simulink model "data_acq_passiveV2"  (R2016b)
settings: Solver=FixedStepDiscrete  StartTime=0.0  StopTime=300  FixedStep=.001  RelTol=1e-3  EnableMultiTasking=on
values from neighbouring files (symbols this model uses):
  offset = [0 0]    [Calibration_Run_Script.m]    (also in DAQ_Run_Script.m; bias.m = signal)
undefined symbols (not defined in the file or in its folder): bit, fdesignblkfcn, gcbh, Standard
libraries: slrtlib x11, xpclib x6, canmsglib x5, simulink x5, xpcnilib x3
(part 2 of 2)

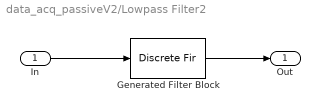
== system data_acq_passiveV2/Lowpass Filter2 ==
  In : Inport
  Generated Filter Block : DiscreteFir  Tag=BlockMethodSubSystem  Coefficients=[0.0035257793515495774 0.0038119531647798038 0.0041036148788394806 0.0044003780267683791 0.0047018389448218933 0.0050075775498282637 0.0053171581667394901 0.0056301304044040169 0.0059460300774376931 0.0062643801719234971 0.0065846918525311708 0.0069064655085147161 0.0072291918359202803 0.0075523529532183957 0.0078754235474644951 0.0081978720479896055 0.008519161824529782 0.008838752406618456 0.0091561007209909322 0.0094706623436844779 0.0097818927634617959 0.010089248653139572 0.010392189145368247 0.010690177109383412 0.010982680425234054 0.011269173251988259 0.011549137286422439 0.011822063008716528 0.012087450911703952 0.012344812710262444 0.01259367252747858 0.012833568054276996 0.013064051679271809 0.013284691585675896 0.013495072812189788 0.013694798274888394 0.013883489747229208 0.014060788795419015 0.014226357666499202 0.014379880126639598 0.014521062247269227 0.014649633136817507 0.014765345615991476 0.014867976834673335 0.014957328828686459 0.015033229014848307 0.015095530622902396 0.015144113063101152 0.015178882228393269 0.015199770730355538 0.015206738068197194 0.015199770730355538 0.015178882228393269 0.015144113063101152 0.015095530622902396 0.015033229014848307 0.014957328828686459 0.014867976834673335 0.014765345615991476 0.014649633136817507 0.014521062247269227 0.014379880126639598 0.014226357666499202 0.014060788795419015 0.013883489747229208 0.013694798274888394 0.013495072812189788 0.013284691585675896 0.013064051679271809 0.012833568054276996 0.01259367252747858 0.012344812710262444 0.012087450911703952 0.011822063008716528 0.011549137286422439 0.011269173251988259 0.010982680425234054 0.010690177109383412 0.010392189145368247 0.010089248653139572 0.0097818927634617959 0.0094706623436844779 0.0091561007209909322 0.008838752406618456 0.008519161824529782 0.0081978720479896055 0.0078754235474644951 0.0075523529532183957 0.0072291918359202803 0.0069064655085147161 0.0065846918525311708 0.0062643801719234971 0.0059460300774376931 0.0056301304044040169 0.0053171581667394901 0.0050075775498282637 0.0047018389448218933 0.0044003780267683791 0.0041036148788394806 0.0038119531647798038 0.0035257793515495774]  InputProcessing=Columns as channels (frame based)
  Out : Outport
  wires:
  In/1 -> Generated Filter Block/1
  Generated Filter Block/1 -> Out/1

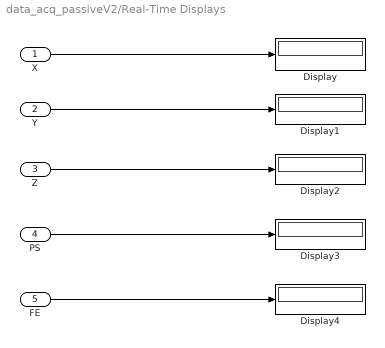
== system data_acq_passiveV2/Real-Time Displays  ==
  X : Inport
  Y : Inport  Port=2
  Z : Inport  Port=3
  PS : Inport  Port=4
  FE : Inport  Port=5
  Display{,1..4} (5 alike) : Display
  wires:
  Y/1 -> Display1/1
  Z/1 -> Display2/1
  PS/1 -> Display3/1
  FE/1 -> Display4/1
  X/1 -> Display/1

== matlab function data_acq_passiveV2/Impedance Control/MATLAB Function ==
  data: tau_m1 output; top input; tau_m2 output; bottom input
function [tau_m1,tau_m2] = f2t(top,bottom)
%#codegen

F1=(top/1901)*(50/.02)*4.4482216;
F2=(bottom/1901)*(50/.02)*4.4482216;

% Ffe = (F1 + F2)/2;
% Ffe = (F1/3) + ((2*F2)/3);
% Fps = (F1 - F2)/2;
% Fps = ((4*F1)/7) - ((3*F2)/7);

%Revision 8/12/14
F1ps=(F1/2.7)-(F2/1.588);
F1fe=(F1+F2)/1.588;
F2ps=(-F1/2.7)+(F2/1.588);
F2fe=(F1+F2)/2.7;

%Revision 9/30/14
% F1ps=(F1-F2)/2;
% F1fe=(F1+F2)/2;
% F2ps=(F2-F1)/2;
% F2fe=(F1+F2)/2;


Ffe=((10*F1fe)+(17*F2fe))/27;
% Ffe=(F1fe+F2fe)/2;
Fps=(F1ps-F2ps)/2;

% tau_m1=Fps/(.76535);
% tau_m2=Ffe/(.8159*2);

tau_m1=Fps*.0435;
tau_m2=Ffe*.065;

% tau_m2 = (.4279*Fps + 1.8251*Ffe - .00755)/(.54395*6);
% tau_m1 = (Fps + 1.9282*Ffe + .18735)/(.41835*3);
% tau_m2 = (1.6738*Fps + 2.9646*Ffe)/(.8936*2);
% tau_m1 = (Fps + 1.1736*Ffe)/(.25815*6);
% tau_m2 = (1.598*Fps + 2.7365*Ffe)/(.8936*3);
% tau_m1 = (Fps + 1.0867*Ffe)/(.2704*3);

% if top > 0 && bottom > 0 %flexion
% %     mA = (bottom + .171786)/.001822;
%     mA = (bottom + .343572)/.003644;

% elseif top > 0 && bottom < 0
%     mA = (bottom - .120011)/-.001265;
%     mA = (bottom - .240022)/-.00253;

% elseif top < 0 && bottom > 0
%     mA = (bottom + .067092)/-.000959;
%     mA = (bottom + .134184)/-.001918;

% elseif top < 0 && bottom < 0 %extension
% %     mA = (bottom - .075747)/.001458;
%     mA = (bottom - .151494)/.002916;
% 
% else 
%     mA = 0;
%     
        
% F2fe=(F1+(.628*F2))/.3157;
% F2ps=F2-F2fe;
% 
% F1fe=-.3123*F2fe;
% F1ps=-.628*F2ps;
% 
% if F2fe > 0
%     tau_fe = -.638*F2fe + .3413;
% elseif F2fe < 0
%     tau_fe = -.7058*F2fe - .1488;
% else
%     tau_fe=0;
% end
% 
% if F2ps > 0
%     tau_ps = 1.1639*F2ps - .3562;
% elseif F2ps < 0
%     tau_ps = .9356*F2ps - .4405;
% else
%     tau_ps=0;
% end
end

== matlab function data_acq_passiveV2/MATLAB Function ==
  data: v1 input; y1 output; v2 input; v3 input; v4 input; v5 input; y2 output; y3 output; y4 output; y5 output; e6 input; e7 input; y6 output; y7 output
function [y1,y2,y3,y4,y5,y6,y7] = volt2deg(v1,v2,v3,v4,v5,e6,e7)
%#codegen

%Enter Calibration Voltages
joint1_zero=8.502;
joint1_25=9.3024;
joint2=4.3443;
joint3_extended=6.6633;
joint3_retracted=0.36838;
joint4=8.8549;
joint5=5.5853;
%-----------------------------------------------
slope1245=(joint1_25 - joint1_zero)/25;
slope3=(joint3_extended - joint3_retracted)/438;

joint1_os=joint1_zero;
joint2_os=joint2 + (slope1245 * 5.6932);
joint4_os=joint4;
joint5_os=joint5;

y1=(joint1_os - v1)./slope1245;
y2=(joint2_os - v2)./slope1245;
y3=(v3 - joint3_retracted)./slope3;
y4=(v4 - joint4_os)./slope1245;
y5=(v5 - joint5_os)./slope1245;
y6=(pi/180)*(30/18750).*e6;
y7=(pi/180)*(30/33920).*e7;

== matlab function data_acq_passiveV2/forward kinematics ==
  data: x output; j1 input; y output; j2 input; d3 input; j4 input; j5 input; j6 input; z output
function [x,y,z] = fcn(j1,j2,d3,j4,j5,j6)
%#codegen

d1=336.55;
a2=434.46;
d4=45.86;
a5=120.51;
d6=67.08;
a6=39.52;

s1=sind(j1);
c1=cosd(j1);
s2=sind(j2);
c2=cosd(j2);
s4=sind(j4);
c4=cosd(j4);
s5=sind(j5);
c5=cosd(j5);
s6=sind(j6);
c6=cosd(j6);

x = -a6*c6*((c1*s2*c5)+s5*((s1*c4)-(c1*c2*s4)))+a6*s6*((s1*s4)+(c1*c2*c4))-d6*((c1*s2*s5)-c5*((s1*c4)-(c1*c2*s4)))-(a5*c1*s2*c5)-a5*s5*((s1*c4)-(c1*c2*s4))-(d4*c1*s2)+((a2+d3)*c1*c2);
y = -a6*c6*((s1*s2*c5)-s5*((c1*c4)+(s1*c2*s4)))-a6*s6*((c1*s4)-(s1*c2*c4))-d6*((s1*s2*s5)+c5*((c1*c4)+(s1*c2*s4)))-(a5*s1*s2*c5)+a5*s5*((c1*c4)+(s1*c2*s4))-(d4*s1*s2)+((a2+d3)*s1*c2);
z = -a6*c6*((c2*c5)+(s2*s4*s5))-(a6*s2*c4*s6)-d6*((c2*s5)-(s2*s4*c5))-(a5*c2*c5)-(a5*s2*s4*s5)-(d4*c2)-((a2+d3)*s2)+d1;

== matlab function data_acq_passiveV2/Impedance Control/MATLAB Function1 ==
  data: current input; signal output; pos input; zero input
function signal = fcn(current,pos,zero)
%#codegen

if pos > -130 && pos < 120
    signal = current;
else
    signal = zero;
end

== matlab function data_acq_passiveV2/Impedance Control/MATLAB Function2 ==
  data: current input; vel input; pos input; signal output
function signal = fcn(current,vel,pos)
%#codegen

% y=exp(-pos.^2/15000);
y=1;
z=1;

if vel >= 3e7
    y=1./(1+exp(-.00000004*vel+4));
elseif vel < -3e7
    y=1./(1+exp(.00000002*vel+3.5));
elseif vel < 3e7 && vel >= -3e7
    y=.05;
end

iscale=current.*y;

if pos >= 0
    z=.9./(1+exp(.0002*pos-8));
elseif pos < 0
    z=.9./(1+exp(-.0002*pos-8));
end

signal=iscale.*z;

end

== matlab function data_acq_passiveV2/Impedance Control/MATLAB Function3 ==
  data: current input; vel input; signal output; pos input
function signal = fcn(current,vel,pos)
%#codegen

% y=exp(-pos.^2/15000);
y=1;
z=1;

if vel >= 3e7
    y=1./(1+exp(-.00000004*vel+4));
elseif vel < -3e7
    y=1./(1+exp(.00000002*vel+3.5));
elseif vel < 3e7 && vel >= -3e7
    y=.05;
end

iscale=current./y;

if pos >= 0
    z=.9./(1+exp(.0002*pos-8));
elseif pos < 0
    z=.9./(1+exp(-.0002*pos-8));
end

signal=iscale./z;

end

== matlab function data_acq_passiveV2/MATLAB Function1 ==
  data: top input; y output; bottom input; clock input
function y = fcn(top,bottom,clock)
%#codegen

stop(data_acq_passiveV2) 
    
ftop=tg.OutputLog(200:end,15);
fbottom=tg.OutputLog(200:end,16);

caltop=mean(ftop);
calbottom=mean(fbottom);

accept=questdlg('Top sensor reads \caltop and bottom sensor reads \calbottom. Proceed with biasing?','Zero Calibration','Yes','No','Yes');
    
    switch accept
        case 'Yes'
            signal=1;
        case 'No'
            signal=0;
    end
y = u;
